simulink model "boiler"  (R2022b)
settings: Solver=ode45  StartTime=0.0  StopTime=ESSettings.tend  RelTol=1e-3  EnableMultiTasking=on
libraries: UtilLib x1
Description:
  | Bang-Bang Control Using Temporal Logic
  | 
  | This example shows how to use Stateflow(R) to model a bang-bang temperature
  | control system for a boiler. The boiler dynamics are modeled in Simulink(R).
  | 
  | The Bang-Bang Controller Stateflow chart shows how to use functions and Subcharts
  | within Stateflow.
settings Model: PacingRate=100  Creator=The MathWorks, Inc.  LastModifiedBy=vd818225
settings SolverCC: AlgebraicLoopSolver=TrustRegion
settings DataIOCC: SaveFormat=Array  SaveOutput=off  SaveTime=off  SignalLoggingName=sigsOut
settings OptimizationCC: BlockReduction=off  BooleanDataType=off  ExpressionDepthLimit=2147483647  InitFltsAndDblsToZero=on  LifeSpan=1  EfficientTunableParamExpr=on
settings DebuggingCC: SaveWithParameterizedLinksMsg=none  UnderspecifiedInitializationDetection=Classic  MergeDetectMultiDrivingBlocksExec=none  SignalResolutionControl=TryResolveAllWithWarning  MultiTaskDSMMsg=warning  MultiTaskCondExecSysMsg=none  FcnCallInpInsideContextMsg=warning  UnconnectedInputMsg=warning  UnconnectedOutputMsg=warning  UnconnectedLineMsg=warning  StateNameClashWarn=warning  SFUnexpectedBacktrackingDiag=warning  SFNoUnconditionalDefaultTransitionDiag=warning  SFExecutionAtInitializationDiag=none  SFMachineParentedDataDiag=warning  ArithmeticOperatorsInVariantConditions=warning
settings HardwareCC: ProdBitPerPointer=32  ProdBitPerSizeT=32  ProdBitPerPtrDiffT=32  ProdLargestAtomicFloat=None  ProdIntDivRoundTo=Undefined  ProdEndianess=Unspecified  ProdWordSize=32  ProdHWDeviceType=ASIC/FPGA  TargetUnknown=on  ProdEqTarget=off
settings ModelReferenceCC: EnableRefExpFcnMdlSchedulingChecks=on  PropagateSignalLabelsOutOfModel=off
settings SFSimCC: SFSimEcho=off  SimUseLocalCustomCode=off  SimParseCustomCode=off  CustomCodeUndefinedFunction=UseInterfaceOnly
settings RTWCC: SystemTargetFile=ert.tlc  GenCodeOnly=on  TemplateMakefile=ert_default_tmf  GenerateReport=on  RTWVerbose=off  RTWUseLocalCustomCode=off  IncludeHyperlinkInReport=on  LaunchReport=on  DLArmComputeVersion=19.05
settings CodeAppCC: IgnoreCustomStorageClasses=off  CustomSymbolStrType=$N$R$M  StateflowObjectComments=on  InternalIdentifier=Classic
settings ERTTargetCC: TargetFcnLib=ansi_tfl_tmw.mat  MultiwordLength=2048  GenerateSampleERTMain=on  SupportContinuousTime=on  SupportNonInlinedSFcns=on  ERTCustomFileTemplate=example_file_process.tlc  ConvertIfToSwitch=off  SuppressUnreachableDefaultCases=off
settings ConfigComp: CovMetricSettings=dcmtr  CovSaveCumulativeToWorkspaceVar=on  CovSaveSingleToWorkspaceVar=on  CovExternalEMLEnable=off

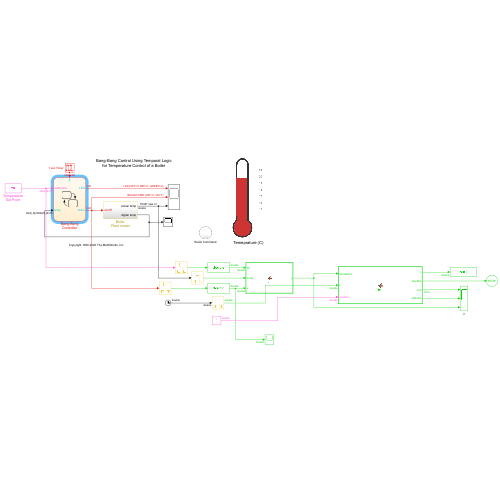
[thumbnail: Simulink's stored preview of the top-level diagram]
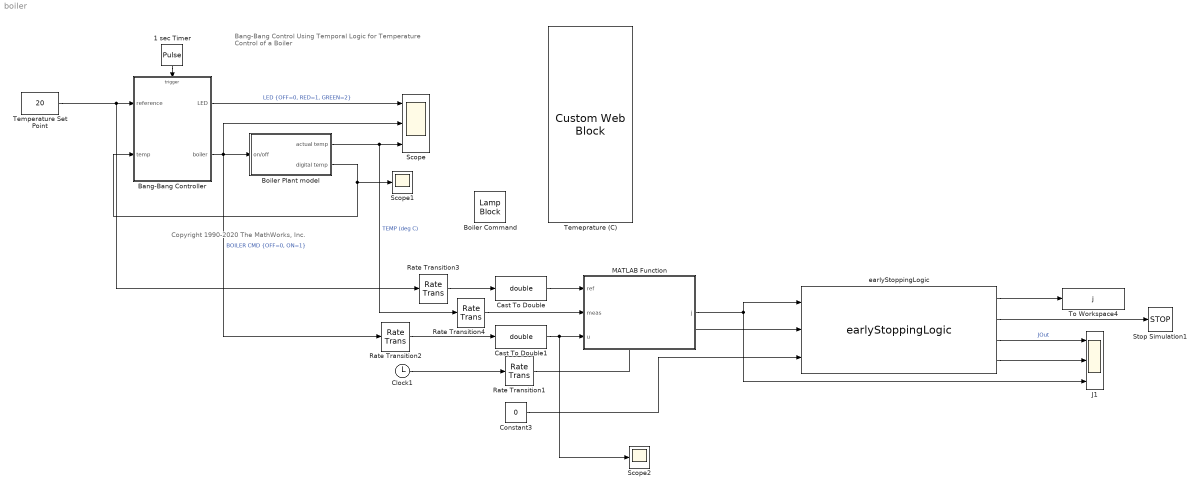
== system boiler ==
  note: Bang-Bang Control Using Temporal Logic
      | for Temperature Control of a Boiler
  note: Copyright 1990-2020 The MathWorks, Inc.
  1 sec Timer : DiscretePulseGenerator  Amplitude=int8(1)
  Bang-Bang Controller : Stateflow chart  TreatAsAtomicUnit=on
  Boiler Plant model : Subsystem
  Boiler Command : LampBlock  LabelPosition=Hide
  Cast To Double : DataTypeConversion  OutDataTypeStr=double  SaturateOnIntegerOverflow=off  RndMeth=Floor
  Cast To Double1 : DataTypeConversion  OutDataTypeStr=double  SaturateOnIntegerOverflow=off  RndMeth=Floor
  Clock1 : Clock
  Constant3 : Constant  Value=0
  J1 : Scope  NumInputPorts=3
  MATLAB Function : MATLAB Function  TreatAsAtomicUnit=on
  Rate Transition{1..4} (4 alike) : RateTransition  OutPortSampleTime=ESSettings.t_obj
  Scope : Scope  NumInputPorts=3
  Scope1 : Scope
  Scope2 : Scope
  Stop Simulation1 : Stop
  Temeprature (C) : CustomWebBlock  LabelPosition=Hide  ShowInitialText=on  Configuration="{\"components\":[{\"name\":\"LinearScaleComponent\",\"settings\":{\"bounds\":{\"max\":22,\"min\":14,\"tickInterval\":1},\"internalTickHeightScaleFactor\":0.5,\"labelColor\":[38,38,38],\"labelFont\":{\"font\":\"Arial\",\"fontSize\":12},\"labelOffset\":0.05,\"labelTransparency\":1,\"needleImage\":{\"size\":[0,0],\"src\":\"\",\"srcOrientation\":\"Right\"},\"needleOffset\":[0,0],\"needleSize\":{\"height\":0,\"width\":0},\"position\":[0.06567112546125461,0.0888569374550683,1.3367361610352264,0.692054889298893],\"referencePoint\":\"auto\",\"scaleColors\":[],\"scaleColorsSize\":0.2,\"scaleDirection\":\"BT\",\"showLabels\":1,\"showMinorTicks\":0,\"showSpanLine\":1,\"showTicks\":1,\"tickColor\":[0,0,0],\"tickTransparency\":0,\"valueBarColor\":[194,0,0],\"valueBarOffset\":0,\"valueBarSize\":0.23,\"valueBarTransparency\":1}},{\"name\":\"BackgroundImageComponent\",\"settings\":{\"image\":{\"size\":[154,384],\"src\":\"data:image\\/svg+xml;base64,PHN2ZyB3aWR0aD0iMTU0IiBoZWlnaHQ9IjM4NCIgeG1sbnM9Imh0dHA6Ly93d3cudzMub3JnLzIwMDAvc3ZnIiB4bWxuczp4bGluaz0iaHR0cDovL3d3dy53My5vcmcvMTk5OS94bGluayIgb3ZlcmZsb3c9ImhpZGRlbiI+PGRlZnM+PGNsaXBQYXRoIGlkPSJjbGlwMCI+PHBhdGggZD0iTTAgMCAxNTQgMCAxNTQgMzg0IDAgMzg0WiIgZmlsbC1ydWxlPSJldmVub2RkIiBjbGlwLXJ1bGU9ImV2ZW5vZGQiLz48L2NsaXBQYXRoPjwvZGVmcz48ZyBjbGlwLXBhdGg9InVybCgjY2xpcDApIj48cmVjdCB4PSIwIiB5PSIwIiB3aWR0aD0i ...(+1892 chars)\",\"srcOrientation\":\"vertical\"},\"position\":[0,0,1,1],\"scaleMode\":\"0\"}},{\"name\":\"ForegroundImageComponent\",\"settings\":{\"image\":{\"size\":[0,0],\"src\":\"default\",\"srcOrientation\":[]},\"isForeground\":1,\"position\":[0,0,1,1],\"scaleMode\":\"0\"}}],\"settings\":{\"BindingType\":\"signal\",\"aspectRatio\":0.4010416666666667,\"backgroundColor\":[0,0,0],\"backgroundOffset\":0,\"backgroundOpacity\":1,\"fixedAspectRatio\":\"on\",\"orientation\":\"vertical\",\"showBackgroundColor\":0,\"version\":\"R2022b\"},\"type\":\"LinearGauge\"}"
  Temperature Set Point : Constant  Value=20  OutDataTypeStr=Inherit: Inherit via back propagation
  To Workspace4 : ToWorkspace  VariableName=j  SaveFormat=Structure With Time  SampleTime=-1
  earlyStoppingLogic : UtilLib/earlyStoppingLogic  SystemSampleTime=-1  VariantActivationTime=update diagram  Latency=0  AutoFrameSizeCalculation=off
  wires:
  1 sec Timer/1 -> Bang-Bang Controller/Trigger
  Bang-Bang Controller/2(boiler) -> Rate Transition2/1, Scope/2, Boiler Plant model/1(on/off)  "BOILER CMD {OFF=0, ON=1}"
  Boiler Plant model/2(digital temp) -> Scope1/1, Bang-Bang Controller/2(temp)
  Boiler Plant model/1(actual temp) -> Rate Transition4/1, Scope/3  "TEMP (deg C)"
  Bang-Bang Controller/1(LED) -> Scope/1  "LED {OFF=0, RED=1, GREEN=2}"
  Constant3/1 -> earlyStoppingLogic/3
  MATLAB Function/1(j) -> earlyStoppingLogic/1, J1/3
  Rate Transition4/1 -> MATLAB Function/2(meas)
  Clock1/1 -> Rate Transition1/1
  Rate Transition3/1 -> Cast To Double/1
  Temperature Set Point/1 -> Rate Transition3/1, Bang-Bang Controller/1(reference)
  Rate Transition1/1 -> earlyStoppingLogic/2
  earlyStoppingLogic/1 -> To Workspace4/1
  earlyStoppingLogic/2 -> Stop Simulation1/1
  earlyStoppingLogic/3 -> J1/1  "JOut"
  earlyStoppingLogic/4 -> J1/2
  Rate Transition2/1 -> Cast To Double1/1
  Cast To Double/1 -> MATLAB Function/1(ref)
  Cast To Double1/1 -> Scope2/1, MATLAB Function/3(u)

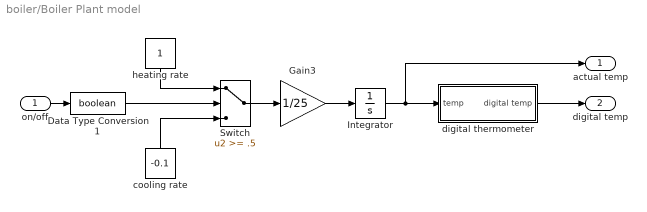
== system boiler/Boiler Plant model ==
  on/off : Inport
  Data Type Conversion1 : DataTypeConversion  OutDataTypeStr=boolean
  Gain3 : Gain  Gain=1/25  SaturateOnIntegerOverflow=on  OutDataTypeStr=Inherit: Same as input  ParamDataTypeStr=Inherit: Same as input
  Integrator : Integrator  InitialCondition=15  ZeroCross=off
  Switch : Switch  Threshold=.5
  cooling rate : Constant  Value=-0.1
  digital thermometer : Subsystem
  heating rate : Constant
  actual temp : Outport  VectorParamsAs1DForOutWhenUnconnected=off
  digital temp : Outport  Port=2  VectorParamsAs1DForOutWhenUnconnected=off
  wires:
  Gain3/1 -> Integrator/1
  cooling rate/1 -> Switch/3
  heating rate/1 -> Switch/1
  Switch/1 -> Gain3/1
  on/off/1 -> Data Type Conversion1/1
  Data Type Conversion1/1 -> Switch/2
  Integrator/1 -> actual temp/1, digital thermometer/1(temp)
  digital thermometer/1(digital temp) -> digital temp/1

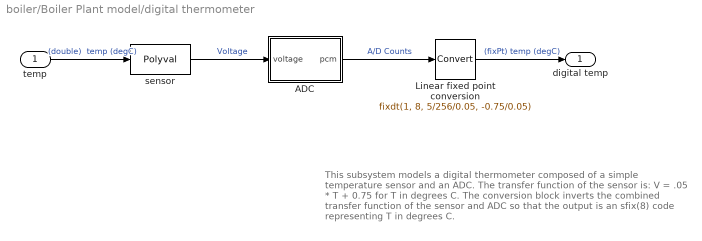
== system boiler/Boiler Plant model/digital thermometer ==
  note: This subsystem models a digital thermometer composed of a simple
      | temperature sensor and an ADC.  The transfer function of the sensor is:
      | V = .05 * T + 0.75
      | for T in degrees C.
      |
      | The conversion block inverts the combined transfer function of the sensor
      | and ADC so that the output is an sfix(8) code representing T in degrees C.
  temp : Inport
  ADC : Subsystem
      mask Display: fprintf('ADC\n8-bit\n0-5V');
  Linear fixed point conversion : DataTypeConversion  OutDataTypeStr=fixdt(1, 8, 5/256/0.05, -0.75/0.05)  ConvertRealWorld=Stored Integer (SI)  SaturateOnIntegerOverflow=off  RndMeth=Floor
  sensor : Polyval  Coefs="[ 0.05     0.75 ]"
  digital temp : Outport  VectorParamsAs1DForOutWhenUnconnected=off
  wires:
  sensor/1 -> ADC/1(voltage)  "Voltage"
  ADC/1(pcm) -> Linear fixed point conversion/1  "A/D Counts"
  temp/1 -> sensor/1  "(double)  temp (degC)"
  Linear fixed point conversion/1 -> digital temp/1  "(fixPt) temp (degC)"

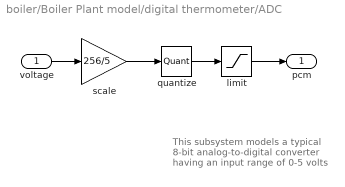
== system boiler/Boiler Plant model/digital thermometer/ADC ==
  note: This subsystem models a typical
      | 8-bit analog-to-digital converter
      | having an input range of 0-5 volts
  voltage : Inport
  limit : Saturate  UpperLimit=255  LowerLimit=0
  quantize : Quantizer  QuantizationInterval=1
  scale : Gain  Gain=256/5  SaturateOnIntegerOverflow=on  OutDataTypeStr=Inherit: Same as input  ParamDataTypeStr=Inherit: Same as input
  pcm : Outport  VectorParamsAs1DForOutWhenUnconnected=off
  wires:
  limit/1 -> pcm/1
  scale/1 -> quantize/1
  quantize/1 -> limit/1
  voltage/1 -> scale/1

== matlab function boiler/MATLAB Function ==
  data: ref input; j output; meas input; u input
function j  = fcn(ref, meas,u)
persistent u_prev

if isempty(u_prev)
    u_prev = 0;
end

comfortSacling = 0.5;

comfort = comfortSacling*(min(abs(ref-meas),2))^2;
energyCost = u;

j = comfort + energyCost;

if u > u_prev
        j =  j + 8;
end

u_prev = u;
end

== stateflow chart boiler/Bang-Bang Controller ==
  state Heater [group]
    state Off
      entry: turn_boiler(OFF)
      on every(5,sec): flash_LED()
    state On
      en: turn_boiler(ON)
      du: flash_LED()
      (history)
      state HIGH
      state NORM
      state b = warm() [function]
        (default) -> (junction 41) : {b = !cold()}
      (default) -> HIGH
      HIGH -> NORM : [warm()]
    (default) -> Off
    On -> Off : after(100,sec)
    Off -> On : after(CtrlPar.TurnOnDelay ,sec)
        | [cold()]
    NORM -> Off : [Heater.On.warm()]
  state turn_boiler(mode) [function]
    (default) -> (junction 32)
    (junction 32) -> (junction 33) [order 1] : [mode==ON]
    (junction 32) -> (junction 43) [order 2] : {color=RED}
    (junction 33) -> (junction 35) : {color=GREEN}
    (junction 43) -> (junction 34)
    (junction 35) -> (junction 34)
    (junction 34) -> (junction 36) : {LED=color;
        |  boiler=mode}
  state flash_LED() [function]
    (default) -> (junction 37)
    (junction 37) -> (junction 38) [order 1] : [LED==OFF]
    (junction 37) -> (junction 31) [order 2] : {LED=OFF}
    (junction 38) -> (junction 42) : {LED=color}
  state b = cold() [function]
    (default) -> (junction 39) : { b = temp<=reference}
  data: b function_output boolean; mode function_input int8; b function_output boolean; LED output int8; boiler output int8; color local int8; reference input fixdt(1,8,1,-15); GREEN constant int8 =2; OFF constant int8; ON constant int8 =1; RED constant int8 =1; temp input fixdt(1,8,0.390625,-15); CtrlPar parameter
  events: sec input RISING_EDGE_EVENT
